simulink model "gain_level_shift"  (R2012b)
settings: Solver=ode45  StartTime=0.0  StopTime=1  RelTol=1e-3
settings Model: Creator=eechris  LastModifiedBy=eechris

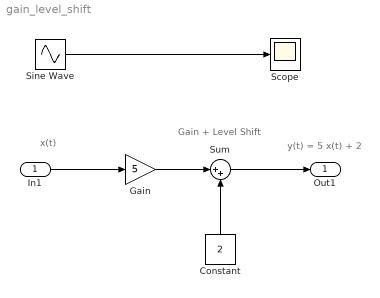
== system gain_level_shift ==
  note: x(t)
  note: y(t) = 5 x(t) + 2
  note: Gain + Level Shift
  In1 : Inport
  Constant : Constant  Value=2
  Gain : Gain  Gain=5
  Scope : Scope
  Sine Wave : Sin  Amplitude=3  Frequency=4*pi  Phase=-3*pi/4  SampleTime=0
  Sum : Sum  Inputs=|++
  Out1 : Outport
  wires:
  Sine Wave/1 -> Scope/1
  Gain/1 -> Sum/1
  Constant/1 -> Sum/2
  In1/1 -> Gain/1
  Sum/1 -> Out1/1
